simulink model "osu_filter"  (R2014b)
settings: Solver=ode45  StartTime=0.0  StopTime=10.0  RelTol=1e-3
undefined symbols (not defined in the file or in its folder): A_lpf_velocity, B1_lpf_velocity, B2_lpf_velocity, initial_hip_roll, initial_torso_pitch, initial_torso_roll, initial_torso_yaw, sample_time, shin_initial_l, shin_initial_r, thigh_initial_l, thigh_initial_r
libraries: simulink x13
settings Model: Creator=xingye  LastModifiedBy=xingye

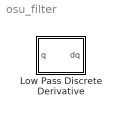
== system osu_filter ==
  Low Pass Discrete Derivative : Subsystem

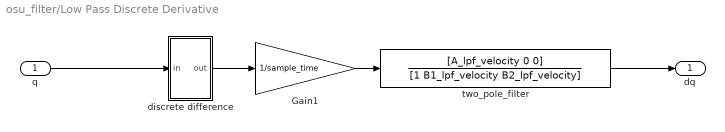
== system osu_filter/Low Pass Discrete Derivative ==
  q : Inport
  Gain1 : Gain  Gain=1/sample_time
  discrete difference : Subsystem
  two_pole_filter : DiscreteTransferFcn  Numerator=[A_lpf_velocity 0 0]  Denominator=[1 B1_lpf_velocity B2_lpf_velocity]  SampleTime=sample_time
  dq : Outport
  wires:
  discrete difference/1(out) -> Gain1/1
  Gain1/1 -> two_pole_filter/1
  two_pole_filter/1 -> dq/1
  q/1 -> discrete difference/1(in)

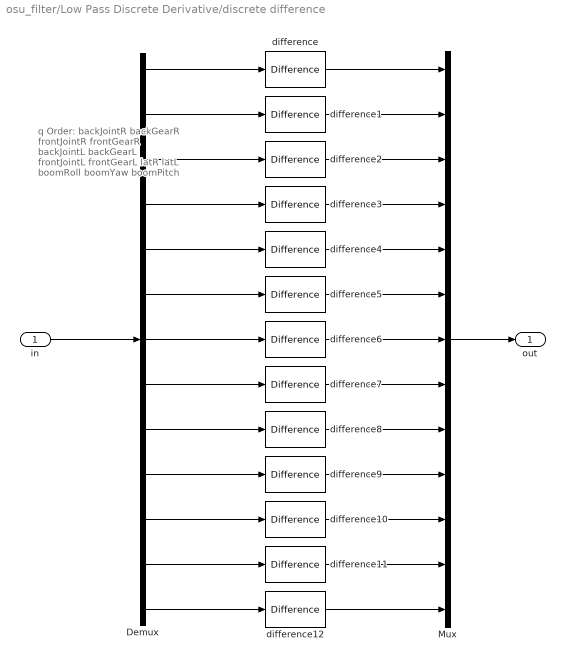
== system osu_filter/Low Pass Discrete Derivative/discrete difference ==
  note: q Order:
      |
      | backJointR
      | backGearR
      | frontJointR
      | frontGearR
      |
      | backJointL
      | backGearL
      | frontJointL
      | frontGearL
      |
      | latR
      | latL
      |
      | boomRoll
      | boomYaw
      | boomPitch
  in : Inport
  Demux : Demux  Outputs=13
  Mux : Mux  Inputs=13
  difference : simulink/Discrete/Difference  ICPrevInput=shin_initial_r  InputProcessing=Columns as channels (frame based)  OutMin=[]  OutMax=[]  OutDataType=fixdt(1, 16)  OutScaling=2^-10  DoSatur=off
  difference1 : simulink/Discrete/Difference  ICPrevInput=shin_initial_r  InputProcessing=Columns as channels (frame based)  OutMin=[]  OutMax=[]  OutDataType=fixdt(1, 16)  OutScaling=2^-10  DoSatur=off
  difference10 : simulink/Discrete/Difference  ICPrevInput=initial_torso_roll  InputProcessing=Columns as channels (frame based)  OutMin=[]  OutMax=[]  OutDataType=fixdt(1, 16)  OutScaling=2^-10  DoSatur=off
  difference11 : simulink/Discrete/Difference  ICPrevInput=initial_torso_yaw  InputProcessing=Columns as channels (frame based)  OutMin=[]  OutMax=[]  OutDataType=fixdt(1, 16)  OutScaling=2^-10  DoSatur=off
  difference12 : simulink/Discrete/Difference  ICPrevInput=initial_torso_pitch  InputProcessing=Columns as channels (frame based)  OutMin=[]  OutMax=[]  OutDataType=fixdt(1, 16)  OutScaling=2^-10  DoSatur=off
  difference2 : simulink/Discrete/Difference  ICPrevInput=thigh_initial_r  InputProcessing=Columns as channels (frame based)  OutMin=[]  OutMax=[]  OutDataType=fixdt(1, 16)  OutScaling=2^-10  DoSatur=off
  difference3 : simulink/Discrete/Difference  ICPrevInput=thigh_initial_r  InputProcessing=Columns as channels (frame based)  OutMin=[]  OutMax=[]  OutDataType=fixdt(1, 16)  OutScaling=2^-10  DoSatur=off
  difference4 : simulink/Discrete/Difference  ICPrevInput=shin_initial_l  InputProcessing=Columns as channels (frame based)  OutMin=[]  OutMax=[]  OutDataType=fixdt(1, 16)  OutScaling=2^-10  DoSatur=off
  difference5 : simulink/Discrete/Difference  ICPrevInput=shin_initial_l  InputProcessing=Columns as channels (frame based)  OutMin=[]  OutMax=[]  OutDataType=fixdt(1, 16)  OutScaling=2^-10  DoSatur=off
  difference6 : simulink/Discrete/Difference  ICPrevInput=thigh_initial_l  InputProcessing=Columns as channels (frame based)  OutMin=[]  OutMax=[]  OutDataType=fixdt(1, 16)  OutScaling=2^-10  DoSatur=off
  difference7 : simulink/Discrete/Difference  ICPrevInput=thigh_initial_l  InputProcessing=Columns as channels (frame based)  OutMin=[]  OutMax=[]  OutDataType=fixdt(1, 16)  OutScaling=2^-10  DoSatur=off
  difference8 : simulink/Discrete/Difference  ICPrevInput=initial_hip_roll  InputProcessing=Columns as channels (frame based)  OutMin=[]  OutMax=[]  OutDataType=fixdt(1, 16)  OutScaling=2^-10  DoSatur=off
  difference9 : simulink/Discrete/Difference  ICPrevInput=initial_hip_roll  InputProcessing=Columns as channels (frame based)  OutMin=[]  OutMax=[]  OutDataType=fixdt(1, 16)  OutScaling=2^-10  DoSatur=off
  out : Outport
  wires:
  difference/1 -> Mux/1
  difference12/1 -> Mux/13
  Demux/13 -> difference12/1
  difference11/1 -> Mux/12
  Demux/12 -> difference11/1
  difference10/1 -> Mux/11
  Demux/11 -> difference10/1
  difference9/1 -> Mux/10
  Demux/10 -> difference9/1
  difference8/1 -> Mux/9
  Demux/9 -> difference8/1
  difference7/1 -> Mux/8
  Demux/8 -> difference7/1
  difference6/1 -> Mux/7
  Demux/7 -> difference6/1
  difference5/1 -> Mux/6
  Demux/6 -> difference5/1
  difference4/1 -> Mux/5
  Demux/5 -> difference4/1
  difference3/1 -> Mux/4
  Demux/4 -> difference3/1
  difference2/1 -> Mux/3
  Demux/3 -> difference2/1
  difference1/1 -> Mux/2
  Demux/2 -> difference1/1
  Mux/1 -> out/1
  in/1 -> Demux/1
  Demux/1 -> difference/1
